simulink model "task3"  (R2023b)
settings: Solver=VariableStepAuto  StartTime=0.0  StopTime=10  MaxStep=0.01  RelTol=1e-4  EnableMultiTasking=on
settings Model: Creator=mitcher  LastModifiedBy=mitcher
settings SolverCC: AlgebraicLoopSolver=TrustRegion
settings DataIOCC: LimitDataPoints=on  SaveOutput=off  SaveTime=off
settings OptimizationCC: ExpressionDepthLimit=2147483647  LifeSpan=1
settings DebuggingCC: UnderspecifiedInitializationDetection=Classic  MergeDetectMultiDrivingBlocksExec=none  FcnCallInpInsideContextMsg=warning  UnconnectedInputMsg=warning  UnconnectedOutputMsg=warning  UnconnectedLineMsg=warning  AllowSymbolicDim=off  StateNameClashWarn=warning  SFUnexpectedBacktrackingDiag=warning  SFNoUnconditionalDefaultTransitionDiag=warning  SFExecutionAtInitializationDiag=none  ArithmeticOperatorsInVariantConditions=warning
settings ModelReferenceCC: EnableRefExpFcnMdlSchedulingChecks=on
settings SFSimCC: SimUseLocalCustomCode=off  CustomCodeUndefinedFunction=UseInterfaceOnly
settings RTWCC: RTWUseLocalCustomCode=off
settings CodeAppCC: StateflowObjectComments=on
settings GRTTargetCC: TargetLangStandard=C89/C90 (ANSI)  CombineOutputUpdateFcns=off  GRTInterface=on

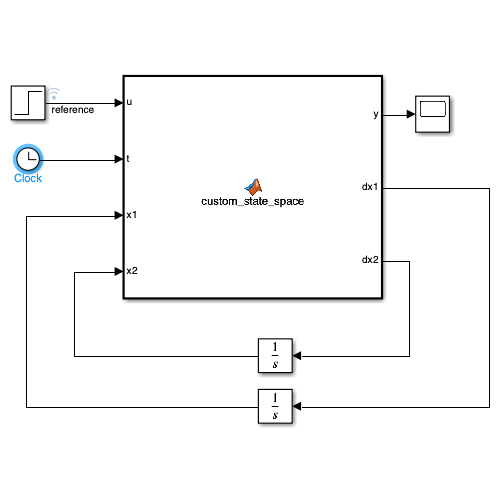
[thumbnail: Simulink's stored preview of the top-level diagram]
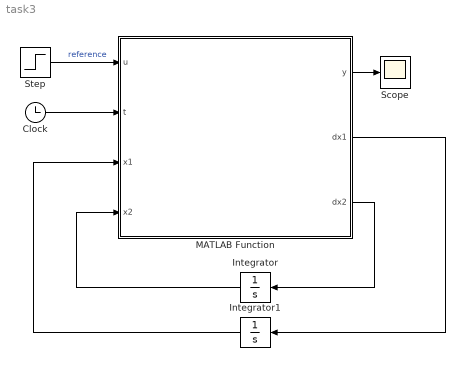
== system task3 ==
  Clock : Clock
  Integrator : Integrator
  Integrator1 : Integrator
  MATLAB Function : MATLAB Function  TreatAsAtomicUnit=on
  Scope : Scope
  Step : Step  SampleTime=0
  wires:
  Step/1 -> MATLAB Function/1(u)  "reference"
  Clock/1 -> MATLAB Function/2(t)
  MATLAB Function/2(dx1) -> Integrator1/1
  MATLAB Function/3(dx2) -> Integrator/1
  Integrator/1 -> MATLAB Function/4(x2)
  Integrator1/1 -> MATLAB Function/3(x1)
  MATLAB Function/1(y) -> Scope/1

== matlab function task3/MATLAB Function ==
  data: u input; y output; t input; x1 input; x2 input; dx1 output; dx2 output
function [y, dx1, dx2] = custom_state_space(u, t, x1, x2)
    dx1 = -4*x1 + x2;
    dx2 = 5*x1-6*sin(t)*x2+3*u;
    y = x1;
